simulink model "ZiemskiAlgorytmPodstawowy"  (R2017a)
settings: Solver=ode113  StartTime=0.0  StopTime=10.0  RelTol=1e-6
values from neighbouring files (symbols this model uses):
  param = evalin('base','param')    [getSaveInfo.m]    (also in loadBackUp.m)
(part 1 of 2)
settings Model: Creator=www  LastModifiedBy=www
settings SolverCC: MaxConsecutiveMinStep=1000  AlgebraicLoopSolver=LineSearch
settings DataIOCC: SaveOutput=off  SignalLogging=off  DSMLogging=off  SaveTime=off

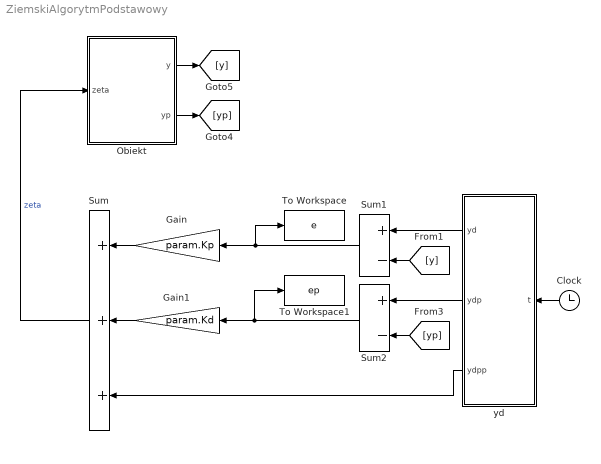
== system ZiemskiAlgorytmPodstawowy ==
  Clock : Clock
  Gain : Gain  Gain=param.Kp
  Gain1 : Gain  Gain=param.Kd
  Obiekt : Subsystem
  Sum : Sum  Inputs=+++
  Sum1 : Sum  Inputs=+-
  Sum2 : Sum  Inputs=+-
  To Workspace : ToWorkspace  VariableName=e  SaveFormat=Timeseries  SampleTime=-1
  To Workspace1 : ToWorkspace  VariableName=ep  SaveFormat=Timeseries  SampleTime=-1
  yd : MATLAB Function  TreatAsAtomicUnit=on
  wires:
  Gain/1 -> Sum/1
  Gain1/1 -> Sum/2
  Sum1/1 -> To Workspace/1, Gain/1
  Obiekt/2(yp) -> [yp]
  Obiekt/1(y) -> [y]
  Sum2/1 -> To Workspace1/1, Gain1/1
  yd/2(ydp) -> Sum2/1
  [yp] -> Sum2/2
  [y] -> Sum1/2
  yd/1(yd) -> Sum1/1
  yd/3(ydpp) -> Sum/3
  Sum/1 -> Obiekt/1(zeta)  "zeta"
  Clock/1 -> yd/1(t)

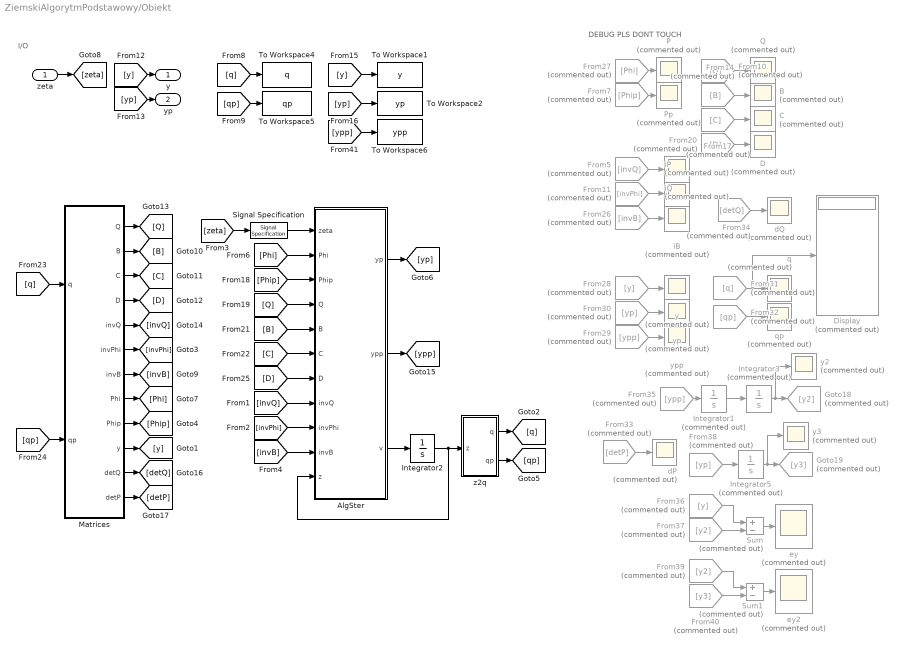
== system ZiemskiAlgorytmPodstawowy/Obiekt ==
  note: I/O
  note: DEBUG PLS DONT TOUCH
  zeta : Inport
  AlgSter : MATLAB Function  TreatAsAtomicUnit=on
  B : Scope  Commented=on
  C : Scope  Commented=on
  D : Scope  Commented=on
  Display : Display  Commented=on
  From10 : From  Commented=on  GotoTag=Q
  From11 : From  Commented=on  GotoTag=invPhi
  From14 : From  Commented=on  GotoTag=B
  From17 : From  Commented=on  GotoTag=C
  From20 : From  Commented=on  GotoTag=D
  From26 : From  Commented=on  GotoTag=invB
  From27 : From  Commented=on  GotoTag=Phi
  From28 : From  Commented=on  GotoTag=y
  From29 : From  Commented=on  GotoTag=ypp
  From30 : From  Commented=on  GotoTag=yp
  From31 : From  Commented=on  GotoTag=q
  From32 : From  Commented=on  GotoTag=qp
  From33 : From  Commented=on  GotoTag=detP
  From34 : From  Commented=on  GotoTag=detQ
  From35 : From  Commented=on  GotoTag=ypp
  From36 : From  Commented=on  GotoTag=y
  From37 : From  Commented=on  GotoTag=y2
  From38 : From  Commented=on  GotoTag=yp
  From39 : From  Commented=on  GotoTag=y2
  From40 : From  Commented=on  GotoTag=y3
  From5 : From  Commented=on  GotoTag=invQ
  From7 : From  Commented=on  GotoTag=Phip
  Goto18 : Goto  Commented=on  GotoTag=y2
  Goto19 : Goto  Commented=on  GotoTag=y3
  Integrator1 : Integrator  Commented=on  InitialCondition=param.initCond.Yp0
  Integrator2 : Integrator  InitialCondition=param.initCond.z0
  Integrator3 : Integrator  Commented=on  InitialCondition=param.initCond.Y0
  Integrator5 : Integrator  Commented=on  InitialCondition=param.initCond.Y0
  Matrices : MATLAB Function  TreatAsAtomicUnit=on
  P : Scope  Commented=on
  Pp : Scope  Commented=on
  Q : Scope  Commented=on
  Signal Specification : SignalSpecification  Dimensions=[5 1]
  Sum : Sum  Commented=on  Inputs=+-
  Sum1 : Sum  Commented=on  Inputs=+-
  To Workspace1 : ToWorkspace  VariableName=y  SaveFormat=Timeseries  SampleTime=-1
  To Workspace2 : ToWorkspace  VariableName=yp  SaveFormat=Timeseries  SampleTime=-1
  To Workspace4 : ToWorkspace  VariableName=q  SaveFormat=Timeseries  SampleTime=-1
  To Workspace5 : ToWorkspace  VariableName=qp  SaveFormat=Timeseries  SampleTime=-1
  To Workspace6 : ToWorkspace  VariableName=ypp  SaveFormat=Timeseries  SampleTime=-1
  dP : Scope  Commented=on
  dQ : Scope  Commented=on
  ey : Scope  Commented=on
  ey2 : Scope  Commented=on
  iB : Scope  Commented=on
  iP : Scope  Commented=on
  iQ : Scope  Commented=on
  q : Scope  Commented=on
  qp : Scope  Commented=on
  "y " : Scope  Commented=on
  y2 : Scope  Commented=on
  y3 : Scope  Commented=on
  "yp " : Scope  Commented=on
  ypp : Scope  Commented=on
  z2q : Subsystem
  y : Outport
  yp : Outport  Port=2
  wires:
  Integrator2/1 -> z2q/1(z), AlgSter/11(z)
  [zeta] -> Signal Specification/1
  [B] -> AlgSter/5(B)
  zeta/1 -> [zeta]
  [Phip] -> AlgSter/3(Phip)
  Signal Specification/1 -> AlgSter/1(zeta)
  [Q] -> AlgSter/4(Q)
  z2q/1(q) -> [q]
  [q] -> To Workspace4/1
  z2q/2(qp) -> [qp]
  [yp] -> yp/1
  [yp] -> To Workspace2/1
  [y] -> To Workspace1/1
  AlgSter/2(ypp) -> [ypp]
  [y] -> y/1
  [qp] -> To Workspace5/1
  AlgSter/1(yp) -> [yp]
  [Phi] -> AlgSter/2(Phi)
  Matrices/9(Phip) -> [Phip]
  Matrices/8(Phi) -> [Phi]
  [q] -> Matrices/1(q)
  [qp] -> Matrices/2(qp)
  Matrices/4(D) -> [D]
  Matrices/3(C) -> [C]
  Matrices/2(B) -> [B]
  Matrices/1(Q) -> [Q]
  Matrices/5(invQ) -> [invQ]
  [C] -> AlgSter/6(C)
  [D] -> AlgSter/7(D)
  [invQ] -> AlgSter/8(invQ)
  AlgSter/3(v) -> Integrator2/1
  Matrices/10(y) -> [y]
  Matrices/6(invPhi) -> [invPhi]
  Matrices/7(invB) -> [invB]
  [invB] -> AlgSter/10(invB)
  [invPhi] -> AlgSter/9(invPhi)
  From10/1 -> Q/1
  From14/1 -> B/1
  From17/1 -> C/1
  From20/1 -> D/1
  From27/1 -> P/1
  From7/1 -> Pp/1
  From5/1 -> iQ/1
  From11/1 -> iP/1
  From26/1 -> iB/1
  From28/1 -> "y "/1
  From30/1 -> "yp "/1
  From29/1 -> ypp/1
  From31/1 -> Display/1, q/1
  From32/1 -> qp/1
  Matrices/11(detQ) -> [detQ]
  Matrices/12(detP) -> [detP]
  From33/1 -> dP/1
  From34/1 -> dQ/1
  Integrator1/1 -> Integrator3/1
  From35/1 -> Integrator1/1
  Integrator3/1 -> y2/1, Goto18/1
  From36/1 -> Sum/1
  From37/1 -> Sum/2
  Sum/1 -> ey/1
  From38/1 -> Integrator5/1
  Integrator5/1 -> y3/1, Goto19/1
  From40/1 -> Sum1/2
  From39/1 -> Sum1/1
  Sum1/1 -> ey2/1
  [ypp] -> To Workspace6/1

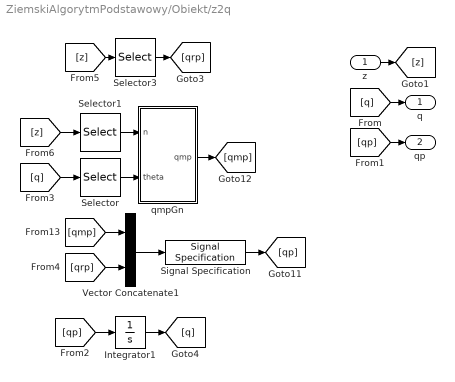
== system ZiemskiAlgorytmPodstawowy/Obiekt/z2q ==
  z : Inport
  Integrator1 : Integrator  InitialCondition=[param.initCond.q0]
  Selector : Selector  InputPortWidth=8  IndexOptions=Index vector (dialog)  Indices=[3]  OutputSizes=1
  Selector1 : Selector  InputPortWidth=5  IndexOptions=Index vector (dialog)  Indices=[1 2]  OutputSizes=1
  Selector3 : Selector  InputPortWidth=5  IndexOptions=Index vector (dialog)  Indices=[3 4 5]  OutputSizes=1
  Signal Specification : SignalSpecification  Dimensions=[8 1]
  Vector Concatenate1 : Concatenate
  qmpGn : MATLAB Function  TreatAsAtomicUnit=on
  q : Outport
  qp : Outport  Port=2
  wires:
  z/1 -> [z]
  [q] -> q/1
  [qp] -> qp/1
  [z] -> Selector1/1
  Selector/1 -> qmpGn/2(theta)
  Selector3/1 -> [qrp]
  [z] -> Selector3/1
  [qp] -> Integrator1/1
  Integrator1/1 -> [q]
  [q] -> Selector/1
  Selector1/1 -> qmpGn/1(n)
  qmpGn/1(qmp) -> [qmp]
  [qmp] -> Vector Concatenate1/1
  [qrp] -> Vector Concatenate1/2
  Vector Concatenate1/1 -> Signal Specification/1
  Signal Specification/1 -> [qp]

== matlab function ZiemskiAlgorytmPodstawowy/Obiekt/z2q/qmpGn ==
  data: n input; qmp output; theta input
function qmp = fcn(n,theta)
L=0.3;
R=0.075;
qmp=[cos(theta), cos(theta);
    sin(theta), sin(theta)
    1/L, -1/L;
    2/R, 0;
    0, 2/R]*n;

== matlab function ZiemskiAlgorytmPodstawowy/Obiekt/AlgSter ==
  data: yp output; ypp output; zeta input; Phi input; Phip input; Q input; B input; C input; D input; invQ input; invPhi input; invB input; z input; v output
function [yp,ypp,v] = fcn(zeta,Phi,Phip,Q,B,C,D,invQ,invPhi,invB,z)

v=invPhi*(-Phip*z+zeta);
%u=invB*(C*z+D+Q*v);
%zp=invQ*(B*u-C*z-D);

yp=Phi*z;
ypp=Phip*z+Phi*v;

== matlab function ZiemskiAlgorytmPodstawowy/yd ==
  data: yd output; ydp output; ydpp output; t input
function [yd,ydp, ydpp] = fcn(t)

% yd=[2*t;
%     0;
%     0.5;
%     -0.3*cos(2*t);
%     0];
% 
% ydp=[2;
%     0;
%     0;
%     0.6*sin(2*t);
%     0];
% 
% ydpp=[0;
%     0;
%     0;
%     1.2*cos(2*t);
%     0];


yd=[2*t;
    -0.3*cos(2*t);
    0.5;
    -0.3;
    0.2];

ydp=[2;
    0.6*sin(2*t);
    0;
    0;
    0];

ydpp=[0;
    1.2*cos(2*t);
    0;
    0;
    0];


% 
% yd=[-0.3*cos(2*t);
%     -0.3*cos(2*t);
%     -0.3*cos(2*t);
%     -0.3*cos(2*t);
%    -0.3*cos(2*t)];
% 
% ydp=[0.6*sin(2*t);
%     0.6*sin(2*t);
%    0.6*sin(2*t);
%     0.6*sin(2*t);
%     0.6*sin(2*t)];
% 
% ydpp=[1.2*cos(2*t);
%     1.2*cos(2*t);
%     1.2*cos(2*t);
%     1.2*cos(2*t);
%     1.2*cos(2*t)];
